simulink library "uavsimBlockset_01to11"  (Simulink 8.0)
settings: Solver=ode45  StartTime=0.0  StopTime=10.0  RelTol=1e-3
settings Model: Creator=mstolle  LastModifiedBy=j.bolting

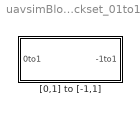
== system uavsimBlockset_01to11 ==
  "[0,1] to [-1,1]" : Subsystem

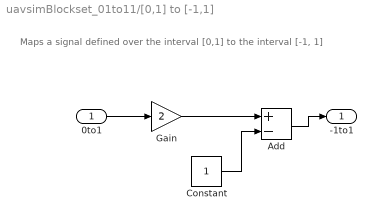
== system uavsimBlockset_01to11/[0,1] to [-1,1] ==
  note: Maps a signal defined over the interval [0,1] to
      | the interval [-1, 1]
  0to1 : Inport
  Add : Sum  Inputs=+-
  Constant : Constant
  Gain : Gain  Gain=2
  -1to1 : Outport
  wires:
  0to1/1 -> Gain/1
  Add/1 -> -1to1/1
  Constant/1 -> Add/2
  Gain/1 -> Add/1
